simulink model "adapt_export"  (Simulink 7.9)
settings: Solver=ode45  StartTime=0.0  StopTime=10.0  RelTol=1e-3
settings Model: Creator=jdenil  LastModifiedBy=jdenil

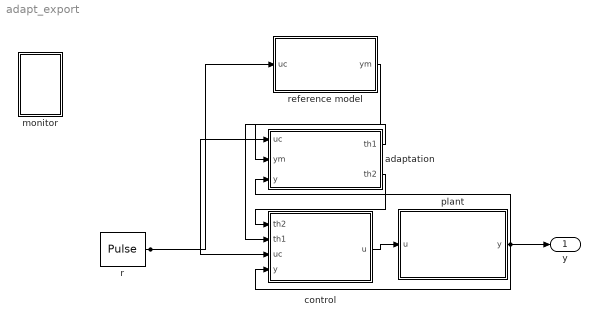
== system adapt_export ==
  adaptation : Subsystem
  control : Subsystem
  monitor : Subsystem
  plant : Subsystem
  r : DiscretePulseGenerator  PulseType=Time based  Amplitude=1.0  Period=20.0  PulseWidth=50.0  PhaseDelay=0.0
  reference model : Subsystem
  y : Outport
  wires:
  adaptation/2(th2) -> control/1(th2)
  adaptation/1(th1) -> control/2(th1)
  plant/1(y) -> control/4(y), adaptation/3(y), y/1
  reference model/1(ym) -> adaptation/2(ym)
  control/1(u) -> plant/1(u)
  r/1 -> control/3(uc), adaptation/1(uc), reference model/1(uc)

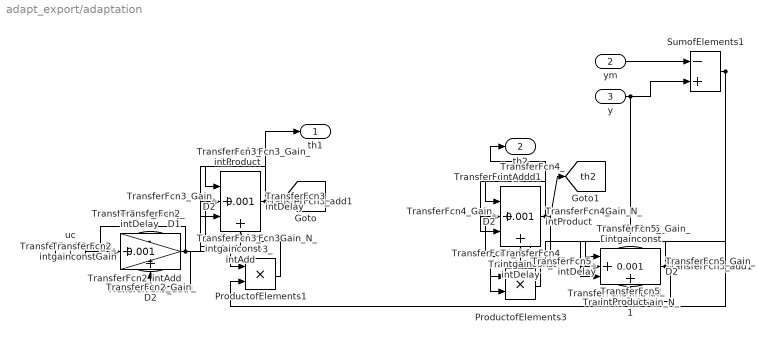
== system adapt_export/adaptation ==
  uc : Inport
  ym : Inport  Port=2
  y : Inport  Port=3
  ProductofElements1 : Product  RndMeth=Zero
  ProductofElements3 : Product  RndMeth=Zero
  SumofElements1 : Sum  Inputs=-+
  TransferFcn2Gain_N_1 : Gain  Gain=3.0
  TransferFcn2_Gain_D1 : Gain  Gain=-3.0
  TransferFcn2_Gain_D2 : Gain  Gain=1.0
  TransferFcn2_add1 : Sum  Inputs=|++
  TransferFcn2_intAdd : Sum  Inputs=|++
  TransferFcn2_intDelay : UnitDelay  SampleTime=0.001
  TransferFcn2_intgainconstGain : Gain  Gain=0.001
  TransferFcn3Gain_N_1 : Gain  Gain=-9.81
  TransferFcn3_Gain_D1 : Gain  Gain=-0.0
  TransferFcn3_Gain_D2 : Gain  Gain=1.0
  TransferFcn3_add1 : Sum  Inputs=|++
  TransferFcn3_intAdd : Sum  Inputs=|++
  TransferFcn3_intDelay : UnitDelay  SampleTime=0.001
  TransferFcn3_intProduct : Product  RndMeth=Zero
  TransferFcn3_intgainconst : Constant  Value=0.001
  TransferFcn4Gain_N_1 : Gain  Gain=9.81
  TransferFcn4_Gain_D1 : Gain  Gain=-0.0
  TransferFcn4_Gain_D2 : Gain  Gain=1.0
  TransferFcn4_add1 : Sum  Inputs=|++
  TransferFcn4_intAdd : Sum  Inputs=|++
  TransferFcn4_intDelay : UnitDelay  SampleTime=0.001
  TransferFcn4_intProduct : Product  RndMeth=Zero
  TransferFcn4_intgainconst : Constant  Value=0.001
  TransferFcn5Gain_N_1 : Gain  Gain=3.0
  TransferFcn5_Gain_D1 : Gain  Gain=-3.0
  TransferFcn5_Gain_D2 : Gain  Gain=1.0
  TransferFcn5_add1 : Sum  Inputs=|++
  TransferFcn5_intAdd : Sum  Inputs=|++
  TransferFcn5_intDelay : UnitDelay  SampleTime=0.001
  TransferFcn5_intProduct : Product  RndMeth=Zero
  TransferFcn5_intgainconst : Constant  Value=0.001
  th1 : Outport
  th2 : Outport  Port=2
  tag scope: th1=global, th2=global
  wires:
  TransferFcn3Gain_N_1/1 -> [th1], th1/1
  ProductofElements1/1 -> TransferFcn3_add1/1
  TransferFcn2Gain_N_1/1 -> ProductofElements1/1
  ym/1 -> SumofElements1/1
  uc/1 -> TransferFcn2_add1/1
  y/1 -> TransferFcn5_add1/1, SumofElements1/2
  SumofElements1/1 -> ProductofElements1/2, ProductofElements3/2
  TransferFcn5Gain_N_1/1 -> ProductofElements3/1
  ProductofElements3/1 -> TransferFcn4_add1/1
  TransferFcn4Gain_N_1/1 -> [th2], th2/1
  TransferFcn4_Gain_D1/1 -> TransferFcn4_add1/2
  TransferFcn4_add1/1 -> TransferFcn4_Gain_D2/1
  TransferFcn4_Gain_D2/1 -> TransferFcn4_intProduct/1
  TransferFcn4_intDelay/1 -> TransferFcn4Gain_N_1/1, TransferFcn4_Gain_D1/1, TransferFcn4_intAdd/2
  TransferFcn3_Gain_D1/1 -> TransferFcn3_add1/2
  TransferFcn3_add1/1 -> TransferFcn3_Gain_D2/1
  TransferFcn3_Gain_D2/1 -> TransferFcn3_intProduct/1
  TransferFcn3_intDelay/1 -> TransferFcn3Gain_N_1/1, TransferFcn3_Gain_D1/1, TransferFcn3_intAdd/2
  TransferFcn5_Gain_D1/1 -> TransferFcn5_add1/2
  TransferFcn5_add1/1 -> TransferFcn5_Gain_D2/1
  TransferFcn5_Gain_D2/1 -> TransferFcn5_intProduct/1
  TransferFcn5_intDelay/1 -> TransferFcn5Gain_N_1/1, TransferFcn5_Gain_D1/1, TransferFcn5_intAdd/2
  TransferFcn2_Gain_D1/1 -> TransferFcn2_add1/2
  TransferFcn2_add1/1 -> TransferFcn2_Gain_D2/1
  TransferFcn2_Gain_D2/1 -> TransferFcn2_intgainconstGain/1
  TransferFcn2_intDelay/1 -> TransferFcn2Gain_N_1/1, TransferFcn2_Gain_D1/1, TransferFcn2_intAdd/2
  TransferFcn2_intgainconstGain/1 -> TransferFcn2_intAdd/1
  TransferFcn2_intAdd/1 -> TransferFcn2_intDelay/1
  TransferFcn5_intgainconst/1 -> TransferFcn5_intProduct/2
  TransferFcn5_intProduct/1 -> TransferFcn5_intAdd/1
  TransferFcn5_intAdd/1 -> TransferFcn5_intDelay/1
  TransferFcn3_intgainconst/1 -> TransferFcn3_intProduct/2
  TransferFcn3_intProduct/1 -> TransferFcn3_intAdd/1
  TransferFcn3_intAdd/1 -> TransferFcn3_intDelay/1
  TransferFcn4_intgainconst/1 -> TransferFcn4_intProduct/2
  TransferFcn4_intProduct/1 -> TransferFcn4_intAdd/1
  TransferFcn4_intAdd/1 -> TransferFcn4_intDelay/1

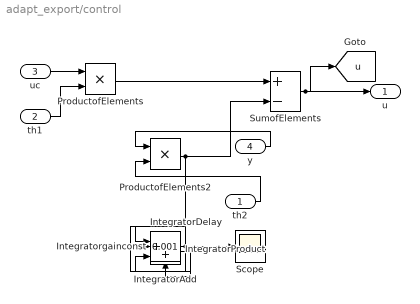
== system adapt_export/control ==
  th2 : Inport
  th1 : Inport  Port=2
  uc : Inport  Port=3
  y : Inport  Port=4
  IntegratorAdd : Sum  Inputs=|++
  IntegratorDelay : UnitDelay  X0=0.0  SampleTime=0.001
  IntegratorProduct : Product  RndMeth=Zero
  Integratorgainconst : Constant  Value=0.001
  ProductofElements : Product  RndMeth=Zero
  ProductofElements2 : Product  RndMeth=Zero
  Scope : Scope
      settings: SaveName=ScopeData2
  SumofElements : Sum  Inputs=+-
  u : Outport
  tag scope: u=global
  wires:
  IntegratorDelay/1 -> Scope/1, IntegratorAdd/2
  th2/1 -> ProductofElements2/2
  SumofElements/1 -> u/1, [u]
  th1/1 -> ProductofElements/2
  y/1 -> ProductofElements2/1
  ProductofElements/1 -> SumofElements/1
  uc/1 -> ProductofElements/1
  ProductofElements2/1 -> SumofElements/2, IntegratorProduct/1
  Integratorgainconst/1 -> IntegratorProduct/2
  IntegratorProduct/1 -> IntegratorAdd/1
  IntegratorAdd/1 -> IntegratorDelay/1

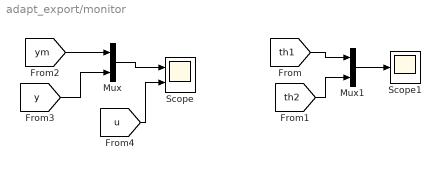
== system adapt_export/monitor ==
  Mux : Mux  Inputs=2
  Mux1 : Mux  Inputs=2
  Scope : Scope  NumInputPorts=2
      settings: SaveName=ScopeData2
  Scope1 : Scope
      settings: SaveName=ScopeData2
  wires:
  [u] -> Scope/2
  [y] -> Mux/2
  [th2] -> Mux1/2
  [ym] -> Mux/1
  Mux1/1 -> Scope1/1
  [th1] -> Mux1/1
  Mux/1 -> Scope/1

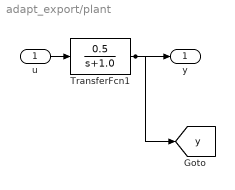
== system adapt_export/plant ==
  u : Inport
  TransferFcn1 : TransferFcn  Numerator=[0.5]  Denominator=[1.0, 1.0]
  y : Outport
  tag scope: y=global
  wires:
  TransferFcn1/1 -> y/1, [y]
  u/1 -> TransferFcn1/1

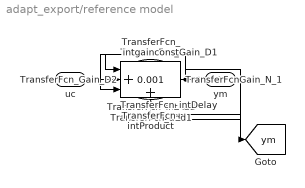
== system adapt_export/reference model ==
  uc : Inport
  TransferFcnGain_N_1 : Gain  Gain=2.0
  TransferFcn_Gain_D1 : Gain  Gain=-3.0
  TransferFcn_Gain_D2 : Gain  Gain=1.0
  TransferFcn_add1 : Sum  Inputs=|++
  TransferFcn_intAdd : Sum  Inputs=|++
  TransferFcn_intDelay : UnitDelay  SampleTime=0.001
  TransferFcn_intProduct : Product  RndMeth=Zero
  TransferFcn_intgainconst : Constant  Value=0.001
  ym : Outport
  tag scope: ym=global
  wires:
  TransferFcnGain_N_1/1 -> ym/1, [ym]
  uc/1 -> TransferFcn_add1/1
  TransferFcn_Gain_D1/1 -> TransferFcn_add1/2
  TransferFcn_add1/1 -> TransferFcn_Gain_D2/1
  TransferFcn_Gain_D2/1 -> TransferFcn_intProduct/1
  TransferFcn_intDelay/1 -> TransferFcnGain_N_1/1, TransferFcn_Gain_D1/1, TransferFcn_intAdd/2
  TransferFcn_intgainconst/1 -> TransferFcn_intProduct/2
  TransferFcn_intProduct/1 -> TransferFcn_intAdd/1
  TransferFcn_intAdd/1 -> TransferFcn_intDelay/1
